simulink model "vdp"  (Simulink 6.0)
settings: Solver=ode45  SolverMode=SingleTasking  StartTime=0.0  StopTime=20  RelTol=1e-3  AbsTol=1e-6
settings Model: Creator=The MathWorks Inc.  LastModifiedBy=batserve  ExtModeAutoUpdateStatusClock=off
settings DataIOCC: ExternalInput=[]  InitialState=[]  LimitDataPoints=off  SaveOutput=off  SaveTime=off
settings OptimizationCC: BlockReduction=off  BooleanDataType=off
settings DebuggingCC: CheckExecutionContextPreStartOutputMsg=on  CheckExecutionContextRuntimeOutputMsg=on  SolverPrmCheckMsg=none
settings HardwareCC: TargetUnknown=on

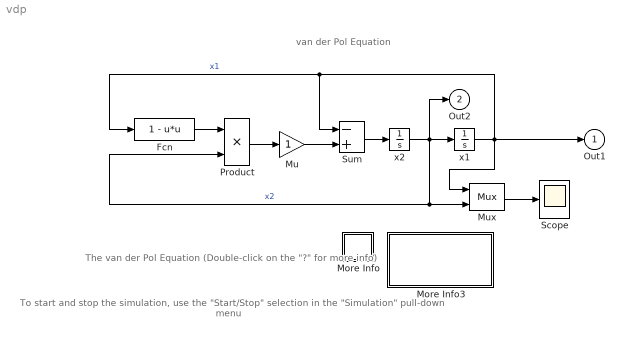
== system vdp ==
  note: van der Pol Equation
  note: To start and stop the simulation, use the "Start/Stop"
      | selection in the "Simulation" pull-down menu
  note: The van der Pol Equation
      | (Double-click on the "?" for more info)
  Fcn : Fcn  Expr=1 - u*u
  More Info : Subsystem  PropExecContextAcrossSSBoundary=on
      mask Display: disp('?')
  More Info3 : Subsystem  PropExecContextAcrossSSBoundary=on
      settings: OpenFcn=simcad(bdroot);
      mask Display: disp('Double-click\nhere for\nSimulink Help')
  Mu : Gain  SaturateOnIntegerOverflow=on
  Mux : Mux  Inputs=2
  Product : Product  SaturateOnIntegerOverflow=on  RndMeth=Zero  InputSameDT=on
  Scope : Scope
      settings: TickLabels=on  TimeRange=20  YMin=-3  YMax=3  DataFormat=Array
  Sum : Sum  Inputs=-+  SaturateOnIntegerOverflow=on  InputSameDT=on
  x1 : Integrator  InitialCondition=2
  x2 : Integrator
  Out1 : Outport  InitialOutput=0
  Out2 : Outport  Port=2  InitialOutput=0
  wires:
  Sum/1 -> x2/1
  x2/1 -> x1/1, Mux/2, Product/2, Out2/1  "x2"
  x1/1 -> Out1/1, Mux/1, Fcn/1, Sum/1  "x1"
  Mux/1 -> Scope/1
  Product/1 -> Mu/1
  Mu/1 -> Sum/2
  Fcn/1 -> Product/1

== system vdp/More Info ==
  note: This demonstration models a second order nonlinear
      | system.
  note: To see a demo of this, just type "vdpdemo" at the
      | command line when the "vdp" window is open.

== system vdp/More Info3 ==
